simulink model "model4_cm"  (R2018b)
settings: Solver=FixedStepDiscrete  StartTime=0.0  StopTime=Inf  FixedStep=0.01  RelTol=1e-3  EnableMultiTasking=on
undefined symbols (not defined in the file): acA2000, Ace, Basler, FreeRun, ipaddr, PoCL, PTP, USETHISONE
libraries: visiontextngfix x10, dotFinder_ul x9, visiongeotforms x1, xpcvideoutillib x1, ptplib x1, rayTrace_ul x1, xpcbitflowlib x1, xpcutilitieslib x1, xpcrtudplib x1
settings Model: sg_rtwmakecfg_data=_bitflow_  SimulationMode=external  Creator=mcobb  LastModifiedBy=mcobb
settings SolverCC: ConcurrentTasks=on  AutoInsertRateTranBlk=on
settings DataIOCC: SaveFormat=StructureWithTime
settings OptimizationCC: BlockReduction=off  OptimizeBlockIOStorage=off  BufferReuse=off  GlobalBufferReuse=off  ExpressionFolding=off  LocalBlockOutputs=off  OptimizeDataStoreBuffers=off  BusAssignmentInplaceUpdate=off
settings DebuggingCC: LibraryContextMissingDiagnostic=none
settings HardwareCC: ProdBitPerPointer=32  ProdBitPerSizeT=32  ProdBitPerPtrDiffT=32  ProdLargestAtomicFloat=None  ProdWordSize=32  ProdLongLongMode=on  ProdHWDeviceType=Generic->32-bit x86 compatible
settings SFSimCC: SimUseLocalCustomCode=off
settings RTWCC: SystemTargetFile=slrt.tlc  TemplateMakefile=slrt_default_tmf  Description=Simulink Real-Time  RTWUseLocalCustomCode=off  CodeExecutionProfiling=on  RTWCompilerOptimization=on
settings SimulinkRealTimeCC: SupportVariableSizeSignals=on  PreserveStateflowLocalDataDimensions=off  RL32ObjectName=tg4  xPCisDefaultEnv=off  xPCTargetPCEnvName=Machine4  xPCConcurrentTasks=on

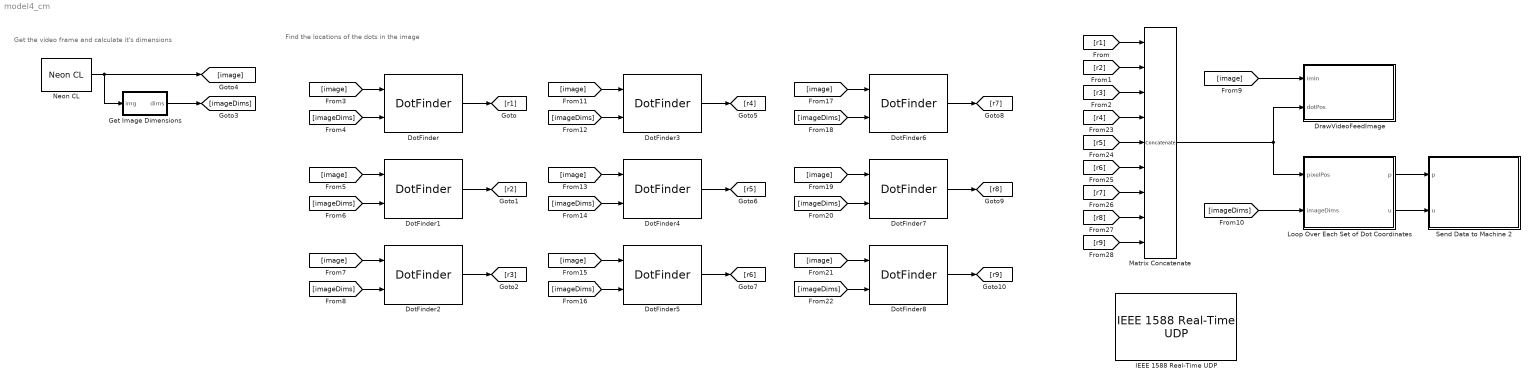
== system model4_cm ==
  note: Get the video frame and calculate it's dimensions
  note: Find the locations of the dots in the image
  DotFinder : dotFinder_ul/DotFinder  ROIPositionHoldEnable=on  ROIPositionHoldCoordinates=[765 998]/3  ROIDimVec_px=[400 100]  ImageDimensions=[1000 2000]
  DotFinder1 : dotFinder_ul/DotFinder  ROIPositionHoldEnable=on  ROIPositionHoldCoordinates=[765 998]/2  ROIDimVec_px=[40 100]  ImageDimensions=[1000 2000]
  DotFinder2 : dotFinder_ul/DotFinder  ROIPositionHoldEnable=on  ROIPositionHoldCoordinates=2*[765 998]/3  ROIDimVec_px=[40 100]  ImageDimensions=[1000 2000]
  DotFinder3 : dotFinder_ul/DotFinder  ROIPositionHoldEnable=on  ROIPositionHoldCoordinates=[765 998]/3  ROIDimVec_px=[400 100]  ImageDimensions=[1000 2000]
  DotFinder4 : dotFinder_ul/DotFinder  ROIPositionHoldEnable=on  ROIPositionHoldCoordinates=[765 998]/2  ROIDimVec_px=[40 100]  ImageDimensions=[1000 2000]
  DotFinder5 : dotFinder_ul/DotFinder  ROIPositionHoldEnable=on  ROIPositionHoldCoordinates=2*[765 998]/3  ROIDimVec_px=[40 100]  ImageDimensions=[1000 2000]
  DotFinder6 : dotFinder_ul/DotFinder  ROIPositionHoldEnable=on  ROIPositionHoldCoordinates=[765 998]/3  ROIDimVec_px=[400 100]  ImageDimensions=[1000 2000]
  DotFinder7 : dotFinder_ul/DotFinder  ROIPositionHoldEnable=on  ROIPositionHoldCoordinates=[765 998]/2  ROIDimVec_px=[40 100]  ImageDimensions=[1000 2000]
  DotFinder8 : dotFinder_ul/DotFinder  ROIPositionHoldEnable=on  ROIPositionHoldCoordinates=2*[765 998]/3  ROIDimVec_px=[40 100]  ImageDimensions=[1000 2000]
  DrawVideoFeedImage : Subsystem
  Get Image Dimensions : Subsystem
  IEEE 1588 Real-Time UDP : ptplib/IEEE 1588 Real-Time UDP  Priority=0  ID=1  PciBus=4  PciSlot=0  PciFunction=0  time_inc=4000000  sample_time=-1  IpSource=Specify  IpAddress=30.30.30.2  SubnetMask=255.255.255.0  Gateway=0.0.0.0  Receive1=30.30.30.30  dest_ip_select=Standard PTP multicast (224.0.1.129, 224.0.0.107)  custom_dest_ip_addr=30.30.30.30  MulticastList=[ipaddr('224.0.1.129'), ipaddr('224.0.0.107')]  Multicast={macaddr('01:00:5E:00:01:81'), macaddr('01:00:5E:00:00:6B')}  time_source=Ethernet board  timescale=PTP (1970-01-01)  epoch=[1970 01 01 00]  delay_measure=Request-response  slave_only=on  enable_advanced_config=on  domain_num=0  utc_offset=35  priority1=128  clock_class=248  clock_accuracy=hex2dec('FE')  priority2=128  announce_interval=1  sync_interval=0.1  min_pdelay_req_interval=2  announce_receipt_timeout=10
      settings: SourceProductName=Simulink Real-Time  SourceProductBaseCode=XP
  Loop Over Each Set of Dot Coordinates : Subsystem  TreatAsAtomicUnit=on
  Matrix Concatenate : Concatenate  NumInputs=9  Mode=Multidimensional array  ConcatenateDimension=2
  "Neon CL " : xpcbitflowlib/Neon CL   camerapath=Basler-Ace-acA2000-340km-E2-PoCL-FreeRun-USETHISONE.r64  r64=CAMERA  sampletime=0.015  slot=-1  make=Basler  model=acA2000-340km  mode=8 bit, 2 tap, 2048x1088, Free Run  owner=BitFlow  revision=1  modelcomp=0  revcomp=0  aqtimeout=4096  format=1  flashmux=Mux_2TOEP  flashdcc=DCC  pixbitdepth=8  xsize=2048  ysize=1088  xstart=0  ystart=0  dx=2048  dy=1088  expmod="[1  0]"  config="[4294967295         128;4294967295           0;4294967295           0;4294967295           0;4294967295           0;4294967295           0;4294967295      262144;4294967295           0;4294967295           0;4294967295           0;4294967295        1024;4294967295           0;4294967295           0;4294967295  4294967295;4294967295           0;4294967295           0;4294967295           0;4294967295      737280;4294967295        1088;4294967295           0;4294967295           0;4294967295           0;4294967295           0;4294967295           0;4294967295           0;4294967295           0;4294967295        7372;4294967295           0]"  ctab="[4      0     16      1   4112      2     16  32768      0]"  qtabmodel="[1   2048  65536]"  trigmode=0  baud=1  bytewidth=4  parity=1  stopbits=1  command="\"\""  response=0  comments=|
      | Free Run Mode / CC Trigger Mode
      | 
      | CC Trigger can be adjusted via GPV0 in CTAB
      | 
      | To use CC Trigger, camera must set to CC Trigger Mode.
      settings: SourceProductName=Simulink Real-Time: Speedgoat I/O Driver Library
  Send Data to Machine 2 : Subsystem
  wires:
  Loop Over Each Set of Dot Coordinates/2(u) -> Send Data to Machine 2/2(u)
  [imageDims] -> DotFinder/2
  DotFinder5/1 -> [r6]
  [image] -> DotFinder2/1
  [r9] -> Matrix Concatenate/9
  DotFinder1/1 -> [r2]
  [r4] -> Matrix Concatenate/4
  [image] -> DotFinder6/1
  [r7] -> Matrix Concatenate/7
  [r6] -> Matrix Concatenate/6
  [image] -> DotFinder8/1
  [image] -> DotFinder/1
  [imageDims] -> DotFinder5/2
  [image] -> DotFinder7/1
  "Neon CL "/1 -> Get Image Dimensions/1(img), [image]
  [imageDims] -> DotFinder6/2
  Loop Over Each Set of Dot Coordinates/1(p) -> Send Data to Machine 2/1(p)
  [r5] -> Matrix Concatenate/5
  [r8] -> Matrix Concatenate/8
  DotFinder6/1 -> [r7]
  [imageDims] -> DotFinder2/2
  [imageDims] -> DotFinder4/2
  [r2] -> Matrix Concatenate/2
  [image] -> DotFinder3/1
  [image] -> DotFinder1/1
  [image] -> DotFinder5/1
  DotFinder8/1 -> [r9]
  [r3] -> Matrix Concatenate/3
  Get Image Dimensions/1(dims) -> [imageDims]
  [imageDims] -> DotFinder1/2
  [image] -> DotFinder4/1
  DotFinder4/1 -> [r5]
  [imageDims] -> DotFinder3/2
  [imageDims] -> Loop Over Each Set of Dot Coordinates/2(imageDims)
  DotFinder7/1 -> [r8]
  Matrix Concatenate/1 -> Loop Over Each Set of Dot Coordinates/1(pixelPos), DrawVideoFeedImage/2(dotPos)
  DotFinder2/1 -> [r3]
  DotFinder/1 -> [r1]
  DotFinder3/1 -> [r4]
  [imageDims] -> DotFinder7/2
  [r1] -> Matrix Concatenate/1
  [imageDims] -> DotFinder8/2
  [image] -> DrawVideoFeedImage/1(imIn)

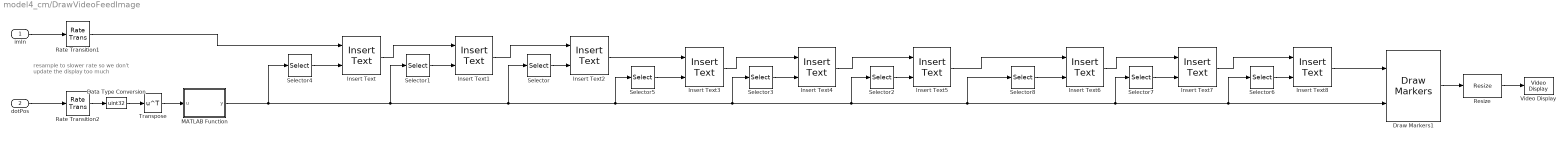
== system model4_cm/DrawVideoFeedImage ==
  note: resample to slower rate so we don't
      | update the display too much
  imIn : Inport
  dotPos : Inport  Port=2
  Data Type Conversion : DataTypeConversion  OutDataTypeStr=uint32
  Draw Markers1 : visiontextngfix/Draw Markers  shape=Circle  size=20  fill=off  fillClrSource=Specify via dialog  display=White  intensity=200  color=[200 255 100]  opacity=0.6  viewport=Entire image  antialiasing=off  inType=Obsolete  imagePorts=One multidimensional signal  prodOutputMode=Binary point scaling  prodOutputWordLength=32  prodOutputFracLength=14  memoryMode=Specify word length  memoryWordLength=16  memoryFracLength=15  roundingMode=Floor  overflowMode=off
      settings: SourceProductName=Computer Vision System Toolbox  SourceProductBaseCode=VP
  Insert Text : visiontextngfix/Insert Text  inputType=Obsolete  theText='1'  getTextLocFrom=Input port  textLoc=[1 1]  getTextColorFrom=Specify via dialog  textColor=255*[1 1 1]  getTextIntensityFrom=Specify via dialog  textIntensity=0  getTextOpacityFrom=Specify via dialog  textOpacity=1.0  dummyVar2=0  dummyVar3=0  dummyVar4=0  imagePorts=One multidimensional signal  isInputTransposed=off  fontFace=LucidaSansRegular  dummyVar1=0  blockFontSize=30  antiAliased=on
      settings: SourceProductName=Computer Vision System Toolbox  SourceProductBaseCode=VP
  Insert Text1 : visiontextngfix/Insert Text  inputType=Obsolete  theText='2'  getTextLocFrom=Input port  textLoc=[1 1]  getTextColorFrom=Specify via dialog  textColor=255*[1 1 1]  getTextIntensityFrom=Specify via dialog  textIntensity=0  getTextOpacityFrom=Specify via dialog  textOpacity=1.0  dummyVar2=0  dummyVar3=0  dummyVar4=0  imagePorts=One multidimensional signal  isInputTransposed=off  fontFace=LucidaSansRegular  dummyVar1=0  blockFontSize=30  antiAliased=on
      settings: SourceProductName=Computer Vision System Toolbox  SourceProductBaseCode=VP
  Insert Text2 : visiontextngfix/Insert Text  inputType=Obsolete  theText='3'  getTextLocFrom=Input port  textLoc=[1 1]  getTextColorFrom=Specify via dialog  textColor=255*[1 1 1]  getTextIntensityFrom=Specify via dialog  textIntensity=0  getTextOpacityFrom=Specify via dialog  textOpacity=1.0  dummyVar2=0  dummyVar3=0  dummyVar4=0  imagePorts=One multidimensional signal  isInputTransposed=off  fontFace=LucidaSansRegular  dummyVar1=0  blockFontSize=30  antiAliased=on
      settings: SourceProductName=Computer Vision System Toolbox  SourceProductBaseCode=VP
  Insert Text3 : visiontextngfix/Insert Text  inputType=Obsolete  theText='4'  getTextLocFrom=Input port  textLoc=[1 1]  getTextColorFrom=Specify via dialog  textColor=255*[1 1 1]  getTextIntensityFrom=Specify via dialog  textIntensity=0  getTextOpacityFrom=Specify via dialog  textOpacity=1.0  dummyVar2=0  dummyVar3=0  dummyVar4=0  imagePorts=One multidimensional signal  isInputTransposed=off  fontFace=LucidaSansRegular  dummyVar1=0  blockFontSize=30  antiAliased=on
      settings: SourceProductName=Computer Vision System Toolbox  SourceProductBaseCode=VP
  Insert Text4 : visiontextngfix/Insert Text  inputType=Obsolete  theText='5'  getTextLocFrom=Input port  textLoc=[1 1]  getTextColorFrom=Specify via dialog  textColor=255*[1 1 1]  getTextIntensityFrom=Specify via dialog  textIntensity=0  getTextOpacityFrom=Specify via dialog  textOpacity=1.0  dummyVar2=0  dummyVar3=0  dummyVar4=0  imagePorts=One multidimensional signal  isInputTransposed=off  fontFace=LucidaSansRegular  dummyVar1=0  blockFontSize=30  antiAliased=on
      settings: SourceProductName=Computer Vision System Toolbox  SourceProductBaseCode=VP
  Insert Text5 : visiontextngfix/Insert Text  inputType=Obsolete  theText='6'  getTextLocFrom=Input port  textLoc=[1 1]  getTextColorFrom=Specify via dialog  textColor=255*[1 1 1]  getTextIntensityFrom=Specify via dialog  textIntensity=0  getTextOpacityFrom=Specify via dialog  textOpacity=1.0  dummyVar2=0  dummyVar3=0  dummyVar4=0  imagePorts=One multidimensional signal  isInputTransposed=off  fontFace=LucidaSansRegular  dummyVar1=0  blockFontSize=30  antiAliased=on
      settings: SourceProductName=Computer Vision System Toolbox  SourceProductBaseCode=VP
  Insert Text6 : visiontextngfix/Insert Text  inputType=Obsolete  theText='7'  getTextLocFrom=Input port  textLoc=[1 1]  getTextColorFrom=Specify via dialog  textColor=255*[1 1 1]  getTextIntensityFrom=Specify via dialog  textIntensity=0  getTextOpacityFrom=Specify via dialog  textOpacity=1.0  dummyVar2=0  dummyVar3=0  dummyVar4=0  imagePorts=One multidimensional signal  isInputTransposed=off  fontFace=LucidaSansRegular  dummyVar1=0  blockFontSize=30  antiAliased=on
      settings: SourceProductName=Computer Vision System Toolbox  SourceProductBaseCode=VP
  Insert Text7 : visiontextngfix/Insert Text  inputType=Obsolete  theText='8'  getTextLocFrom=Input port  textLoc=[1 1]  getTextColorFrom=Specify via dialog  textColor=255*[1 1 1]  getTextIntensityFrom=Specify via dialog  textIntensity=0  getTextOpacityFrom=Specify via dialog  textOpacity=1.0  dummyVar2=0  dummyVar3=0  dummyVar4=0  imagePorts=One multidimensional signal  isInputTransposed=off  fontFace=LucidaSansRegular  dummyVar1=0  blockFontSize=30  antiAliased=on
      settings: SourceProductName=Computer Vision System Toolbox  SourceProductBaseCode=VP
  Insert Text8 : visiontextngfix/Insert Text  inputType=Obsolete  theText='9'  getTextLocFrom=Input port  textLoc=[1 1]  getTextColorFrom=Specify via dialog  textColor=255*[1 1 1]  getTextIntensityFrom=Specify via dialog  textIntensity=0  getTextOpacityFrom=Specify via dialog  textOpacity=1.0  dummyVar2=0  dummyVar3=0  dummyVar4=0  imagePorts=One multidimensional signal  isInputTransposed=off  fontFace=LucidaSansRegular  dummyVar1=0  blockFontSize=30  antiAliased=on
      settings: SourceProductName=Computer Vision System Toolbox  SourceProductBaseCode=VP
  MATLAB Function : MATLAB Function  TreatAsAtomicUnit=on
  Rate Transition1 : RateTransition  Deterministic=off  OutPortSampleTime=5*0.015
  Rate Transition2 : RateTransition  Deterministic=off  OutPortSampleTime=5*0.015
  Resize : visiongeotforms/Resize  specify=Number of output columns and preserve aspect ratio  rfactor=[200 150]  outCols=1000  outRows=25  outRowsCols=[25 35]  interp_method=Bilinear  antialias=on  useROI=off  roiFlag=off  prodOutputMode=Binary point scaling  prodOutputWordLength=32  prodOutputFracLength=10  roundingMode=Nearest  overflowMode=on
      settings: SourceProductName=Computer Vision System Toolbox  SourceProductBaseCode=VP
  Selector : Selector  NumberOfDimensions=2  InputPortWidth=3  IndexOptions=Index vector (dialog),Select all  Indices=3,1  OutputSizes=1,1
  Selector1 : Selector  NumberOfDimensions=2  InputPortWidth=3  IndexOptions=Index vector (dialog),Select all  Indices=2,1  OutputSizes=1,1
  Selector2 : Selector  NumberOfDimensions=2  InputPortWidth=3  IndexOptions=Index vector (dialog),Select all  Indices=6,1  OutputSizes=1,1
  Selector3 : Selector  NumberOfDimensions=2  InputPortWidth=3  IndexOptions=Index vector (dialog),Select all  Indices=5,1  OutputSizes=1,1
  Selector4 : Selector  NumberOfDimensions=2  InputPortWidth=3  IndexOptions=Index vector (dialog),Select all  Indices=1,1  OutputSizes=1,1
  Selector5 : Selector  NumberOfDimensions=2  InputPortWidth=3  IndexOptions=Index vector (dialog),Select all  Indices=4,1  OutputSizes=1,1
  Selector6 : Selector  NumberOfDimensions=2  InputPortWidth=3  IndexOptions=Index vector (dialog),Select all  Indices=9,1  OutputSizes=1,1
  Selector7 : Selector  NumberOfDimensions=2  InputPortWidth=3  IndexOptions=Index vector (dialog),Select all  Indices=8,1  OutputSizes=1,1
  Selector8 : Selector  NumberOfDimensions=2  InputPortWidth=3  IndexOptions=Index vector (dialog),Select all  Indices=7,1  OutputSizes=1,1
  Transpose : Math  Operator=transpose  SaturateOnIntegerOverflow=on
  Video Display : xpcvideoutillib/Video Display  imagesignal=Single multidimensional signal  colorspace=RGB  vindex=1  showpreview=on
      settings: SourceProductName=Simulink Real-Time  SourceProductBaseCode=XP
  wires:
  MATLAB Function/1(y) -> Selector/1, Selector5/1, Selector3/1, Selector2/1, Selector8/1, Selector7/1, Selector6/1, Draw Markers1/2, Selector1/1, Selector4/1
  Rate Transition2/1 -> Data Type Conversion/1
  Rate Transition1/1 -> Insert Text/1
  Data Type Conversion/1 -> Transpose/1
  Insert Text/1 -> Insert Text1/1
  Insert Text1/1 -> Insert Text2/1
  Transpose/1 -> MATLAB Function/1(u)
  Selector1/1 -> Insert Text1/2
  Selector4/1 -> Insert Text/2
  dotPos/1 -> Rate Transition2/1
  Selector/1 -> Insert Text2/2
  imIn/1 -> Rate Transition1/1
  Draw Markers1/1 -> Resize/1
  Resize/1 -> Video Display/1
  Selector2/1 -> Insert Text5/2
  Selector5/1 -> Insert Text3/2
  Selector3/1 -> Insert Text4/2
  Insert Text4/1 -> Insert Text5/1
  Insert Text3/1 -> Insert Text4/1
  Insert Text6/1 -> Insert Text7/1
  Insert Text7/1 -> Insert Text8/1
  Selector7/1 -> Insert Text7/2
  Selector8/1 -> Insert Text6/2
  Selector6/1 -> Insert Text8/2
  Insert Text8/1 -> Draw Markers1/1
  Insert Text2/1 -> Insert Text3/1
  Insert Text5/1 -> Insert Text6/1

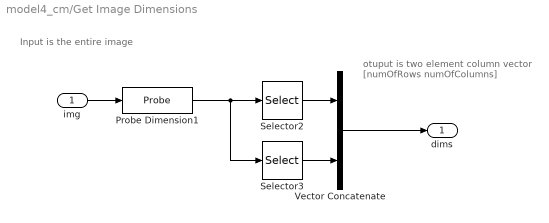
== system model4_cm/Get Image Dimensions ==
  note: otuput is two element column vector
      | [numOfRows numOfColumns]
  note: Input is the entire image
  img : Inport
  Probe Dimension1 : Probe  ProbeWidth=off  ProbeSampleTime=off  ProbeComplexSignal=off  ProbeSignalDimensions=on
  Selector2 : Selector  InputPortWidth=2  IndexOptions=Index vector (dialog)  Indices=1  OutputSizes=1
  Selector3 : Selector  InputPortWidth=2  IndexOptions=Index vector (dialog)  Indices=2  OutputSizes=1
  Vector Concatenate : Concatenate
  dims : Outport
  wires:
  Selector2/1 -> Vector Concatenate/1
  Vector Concatenate/1 -> dims/1
  Probe Dimension1/1 -> Selector2/1, Selector3/1
  Selector3/1 -> Vector Concatenate/2
  img/1 -> Probe Dimension1/1

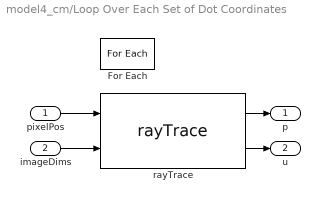
== system model4_cm/Loop Over Each Set of Dot Coordinates ==
  pixelPos : Inport  Partition=on  PartitionDimension=2  PartitionWidth=1  PartitionOffset=0
  imageDims : Inport  Port=2
  For Each : ForEach  DisableCoverage=on  IndexMode=One-based
  rayTrace : rayTrace_ul/rayTrace  camPosVec_cm=[5 0 0]  camEulAngles_deg=[0 90 0]  dist2Glass_cm=1  indOfRefVec=[1 1 1]  glassNormalVec=[1 0 0]  glassThickness_cm=0.1  camFOV_deg=[20 20]
  p : Outport  ConcatenationDimension=2
  u : Outport  Port=2  ConcatenationDimension=2
  wires:
  pixelPos/1 -> rayTrace/1
  rayTrace/1 -> p/1
  rayTrace/2 -> u/1
  imageDims/1 -> rayTrace/2

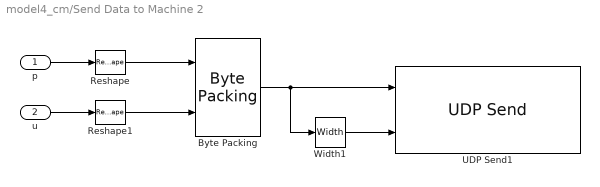
== system model4_cm/Send Data to Machine 2 ==
  p : Inport
  u : Inport  Port=2
  Byte Packing : xpcutilitieslib/Byte Packing   MaskPackedDataType=uint8  MaskUnpackedDataTypes={['double'],['double']}  MaskAlignment=1
  Reshape : Reshape
  Reshape1 : Reshape
  UDP Send1 : xpcrtudplib/UDP Send  ipAddressVal=30.30.30.2  localPort=-1  toAddress=30.30.30.30  toPort=8002  sampleTime=-1
      settings: SourceProductName=Simulink Real-Time  SourceProductBaseCode=XP
  Width1 : Width
  wires:
  p/1 -> Reshape/1
  Reshape1/1 -> Byte Packing/2
  Reshape/1 -> Byte Packing/1
  Byte Packing/1 -> UDP Send1/1, Width1/1
  u/1 -> Reshape1/1
  Width1/1 -> UDP Send1/2

== matlab function model4_cm/DrawVideoFeedImage/MATLAB Function ==
  data: u input; y output
function y = fcn(u)
y = u;
y(:,1) = u(:,2);
y(:,2) = u(:,1);
